simulink model "ams_ut"  (Simulink 8.1)
settings: Solver=FixedStepDiscrete  StartTime=0.0  StopTime=Inf  FixedStep=0.005  RelTol=1e-3
PostLoadFcn:
  | , if any(exist('dsrtsu_mdlpostloadfcn', 'file') == [2, 3, 6]), try dsrtsu_mdlpostloadfcn('Execute', bdroot); catch fprintf('Error in PostLoadFcn (dsrtsu_mdlpostloadfcn) for model "%s":\n %s\n', bdroot, lasterr); end, end,
libraries: siltestlib x7, ams x1
settings Model: DSRTSU_INTERNAL_RTI_VER=450  DSRTSU_INTERNAL_RTI_TYPE=rti1401  RTICANMMDATA=struct('GeneralSetupData',struct('modelroot','D:\ELN150201_TAIWAN\trunk\AdasDragon\software\sw_development\arch\app\ifo','generalsettings',struct('filesettings',struct('destfolder',struct('Name','RTICANMM_FILES','Check',1),'buildfolder',struct('Name','.','Check',1),'AbsDestfolder',struct('Name','D:\ELN150201_TAIWAN\trunk\AdasDragon\software\sw_development\arch\app\ifo\RTICANMM_FILES'),'AbsBuildfolder',struct('Name','D:\ELN150201_TAIWAN\trunk\AdasDragon\software\sw_development\arch\app\ifo'))),'options',struct('addpaths',1,'rmpaths',1,'addtrcexclusion',logical(1),'cannavigator',struct('checkmonitoring',0),'show_usrtrc',0,'use_usrtrc',0),'advanced',struct('options',[1 1 1 1 1 1 1 1 1 1 1 1 1 1 1 1 1 1 1 1 1 1 1 1 1 1 1 1 1 1 1 1 1 1 1 1 1 1 1 1 1 1 1 1 1 1 1 1 1 1 1 1 1 1 1 1 1 1 1 1 1 1 1 1 1 1 1 1 1 1 1 1 1 1 1 1 1 1 1 1 1 1 1 1 1 1 1 1 1 1 1 1 1 1 1 1 1 1 1 1]),'MPSetup',{{}},'modelname','ams_ut','block','ams_ut'))  DSRTSU_INTERNAL_RTIFPGA=40  Creator=AT015411  LastModifiedBy=AT015555  BufferReuse=off
settings DataIOCC: SignalLoggingSaveFormat=Dataset
settings OptimizationCC: BlockReduction=off  OptimizeBlockIOStorage=off  BufferReuse=off  ExpressionFolding=off  ExpressionDepthLimit=128  LocalBlockOutputs=off
settings DebuggingCC: FcnCallInpInsideContextMsg=EnableAllAsError
settings HardwareCC: ProdIntDivRoundTo=Zero  ProdEndianess=BigEndian  ProdHWDeviceType=Generic->Custom  TargetIntDivRoundTo=Zero  TargetEndianess=BigEndian  TargetHWDeviceType=Generic->Custom
settings RTWCC: SystemTargetFile=rti1005.tlc  MakeCommand=make_rti  TemplateMakefile=rti1005.tmf  Description=dSPACE DS1005 Hardware Platform  ProcessScript=rti1005_make_rtw_hook
settings STFCustomTargetCC: CodeReplacementLibrary=ANSI_C  ParMdlRefBuildCompliant=on  GeneratePreprocessorConditionals=Disable all  MatFileLogging=on  SystemTargetFile=rti1005.tlc
settings GRTTargetCC: CompOptLevelCompliant=off  ConcurrentExecutionCompliant=off  ExtModeMexFile=noextcomm
settings CustomProperty: DataType=RTWOptions_EnumType_C__Program Files (x86)_dSPACE RCPHIL 2014-B_MATLAB_RTI_RTI1401_TLC_rti1005_1InitialSimState  Value=RUN
settings EnumStrPairs: String=RUN

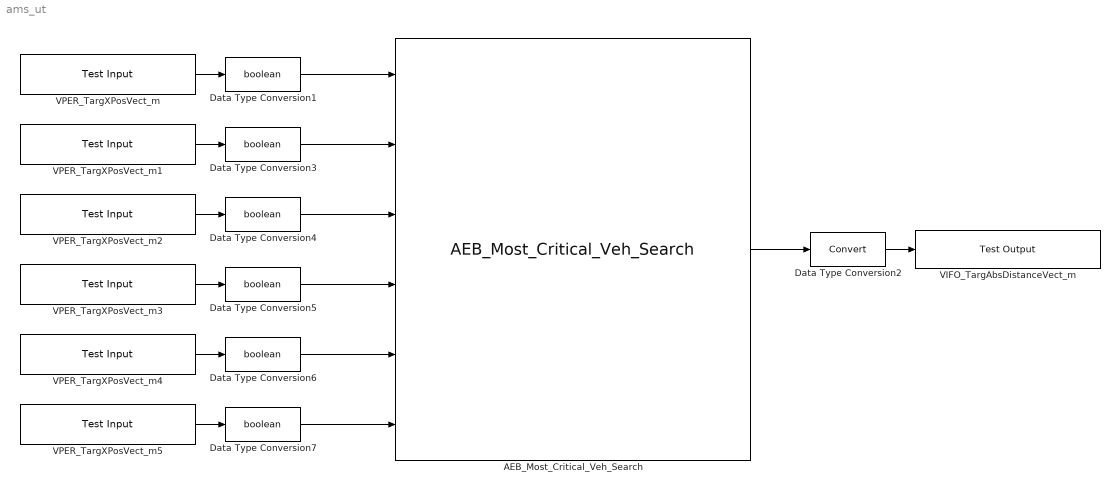
== system ams_ut ==
  AEB_Most_Critical_Veh_Search : ams/AEB_Most_Critical_Veh_Search
  Data Type Conversion{1,3..7} (6 alike) : DataTypeConversion  OutDataTypeStr=boolean
  Data Type Conversion2 : DataTypeConversion
  VIFO_TargAbsDistanceVect_m : siltestlib/Test Output  varname=VIFO_AEBMCTTargId_num  sampletime=-1
  VPER_TargXPosVect_m : siltestlib/Test Input  varname=NIFO_TargetNIsVeh_flg  sampletime=0.005
  VPER_TargXPosVect_m1 : siltestlib/Test Input  varname=NIFO_TargetNSameDir_flg  sampletime=0.005
  VPER_TargXPosVect_m2 : siltestlib/Test Input  varname=NIFO_VehicleNInPathAEB_flg  sampletime=0.005
  VPER_TargXPosVect_m3 : siltestlib/Test Input  varname=NIFO_TargNAbsDistance_m  sampletime=0.005
  VPER_TargXPosVect_m4 : siltestlib/Test Input  varname=NIFO_TargetNExistProb_num  sampletime=0.005
  VPER_TargXPosVect_m5 : siltestlib/Test Input  varname=NIFO_IterationN_enum  sampletime=0.005
  wires:
  VPER_TargXPosVect_m/1 -> Data Type Conversion1/1
  Data Type Conversion1/1 -> AEB_Most_Critical_Veh_Search/1
  AEB_Most_Critical_Veh_Search/1 -> Data Type Conversion2/1
  Data Type Conversion2/1 -> VIFO_TargAbsDistanceVect_m/1
  VPER_TargXPosVect_m1/1 -> Data Type Conversion3/1
  Data Type Conversion3/1 -> AEB_Most_Critical_Veh_Search/2
  VPER_TargXPosVect_m2/1 -> Data Type Conversion4/1
  Data Type Conversion4/1 -> AEB_Most_Critical_Veh_Search/3
  VPER_TargXPosVect_m3/1 -> Data Type Conversion5/1
  Data Type Conversion5/1 -> AEB_Most_Critical_Veh_Search/4
  VPER_TargXPosVect_m4/1 -> Data Type Conversion6/1
  Data Type Conversion6/1 -> AEB_Most_Critical_Veh_Search/5
  VPER_TargXPosVect_m5/1 -> Data Type Conversion7/1
  Data Type Conversion7/1 -> AEB_Most_Critical_Veh_Search/6
